simulink model "nl_cart_5"  (R2022a)
settings: Solver=ode45  StartTime=0.0  StopTime=40  MaxStep=0.001  MinStep=0.000001  RelTol=1e-3
values from neighbouring files (symbols this model uses):
  b = 1    [ex4.m]
  dth0 = 0    [ex4.m]
  dx0 = 0    [ex4.m]
  g = 9.81    [ex4.m]
  Ie = I + m * l^2    (= 0.02603525)    [ex4.m]
  l = 0.305    [ex4.m]
  m = 0.21    [ex4.m]
  Me = M + m    (= 0.665)    [ex4.m]
  th0 = pi / 6    (= 0.523598775598)    [ex4.m]
  x0 = 0    [ex4.m]
undefined symbols (not defined in the file or in its folder): d, denth, denx, numth, numx, st
settings Model: Creator=loren  LastModifiedBy=loren
settings DataIOCC: ReturnWorkspaceOutputs=off

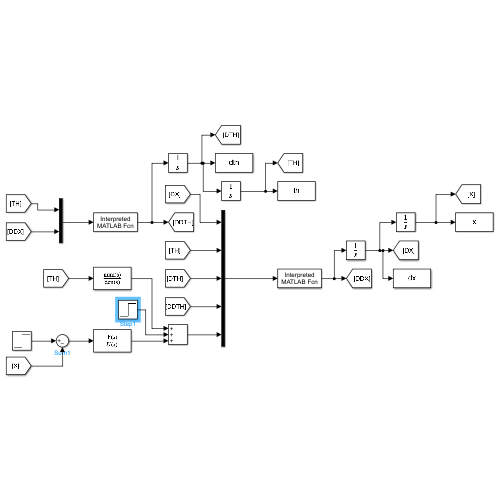
[thumbnail: Simulink's stored preview of the top-level diagram]
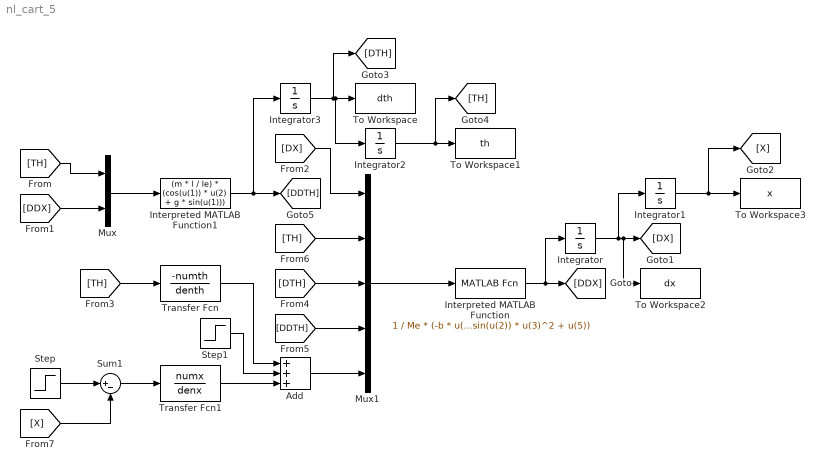
== system nl_cart_5 ==
  Add : Sum  Inputs=+++
  Integrator : Integrator  InitialCondition=dx0
  Integrator1 : Integrator  InitialCondition=x0
  Integrator2 : Integrator  InitialCondition=th0
  Integrator3 : Integrator  InitialCondition=dth0
  Interpreted MATLAB Function : MATLABFcn  MATLABFcn=1 / Me * (-b * u(1) + m * l * cos(u(2)) * u(4) - m * l * sin(u(2)) * u(3)^2 + u(5))  OutputDimensions=1
  Interpreted MATLAB Function1 : MATLABFcn  MATLABFcn=(m * l / Ie) * (cos(u(1)) * u(2) + g * sin(u(1)))  OutputDimensions=1
  Mux : Mux  Inputs=2
  Mux1 : Mux  Inputs=5
  Step : Step  Time=st.t  After=st.A  SampleTime=0
  Step1 : Step  Time=d.t  After=d.A  SampleTime=0
  Sum1 : Sum  Inputs=|+-
  To Workspace : ToWorkspace  VariableName=dth  SaveFormat=Timeseries  SampleTime=-1
  To Workspace1 : ToWorkspace  VariableName=th  SaveFormat=Timeseries  SampleTime=-1
  To Workspace2 : ToWorkspace  VariableName=dx  SaveFormat=Timeseries  SampleTime=-1
  To Workspace3 : ToWorkspace  VariableName=x  SaveFormat=Timeseries  SampleTime=-1
  Transfer Fcn : TransferFcn  Numerator=-numth  Denominator=denth
  Transfer Fcn1 : TransferFcn  Numerator=numx  Denominator=denx
  wires:
  Sum1/1 -> Transfer Fcn1/1
  Step1/1 -> Add/2
  Step/1 -> Sum1/1
  Transfer Fcn1/1 -> Add/3
  [TH] -> Transfer Fcn/1
  [X] -> Sum1/2
  [DX] -> Mux1/1
  Add/1 -> Mux1/5
  Transfer Fcn/1 -> Add/1
  [DDTH] -> Mux1/4
  Mux/1 -> Interpreted MATLAB Function1/1
  Mux1/1 -> Interpreted MATLAB Function/1
  [DTH] -> Mux1/3
  [TH] -> Mux1/2
  [DDX] -> Mux/2
  [TH] -> Mux/1
  Interpreted MATLAB Function1/1 -> Integrator3/1, [DDTH]
  Interpreted MATLAB Function/1 -> Integrator/1, [DDX]
  Integrator/1 -> To Workspace2/1, [DX], Integrator1/1
  Integrator3/1 -> To Workspace/1, Integrator2/1, [DTH]
  Integrator1/1 -> To Workspace3/1, [X]
  Integrator2/1 -> To Workspace1/1, [TH]
